simulink model "SEIRS_2_Control_Filtro"  (R2024a)
settings: Solver=VariableStepAuto  StartTime=0.0  StopTime=Dias  RelTol=1e-3
model workspace (MAT data in the model file):
  x = [0.0844291205376 0.0972801431163 0.171504041231 0.000911075297271]
undefined symbols (not defined in the file): I0, K_control, pert, R0, S0, Ts, TS, u_0, x0
libraries: simulink x1
settings Model: Creator=carlo  LastModifiedBy=luism
settings DataIOCC: SaveOutput=off
settings RTWCC: GPUComputeCapability=3.5

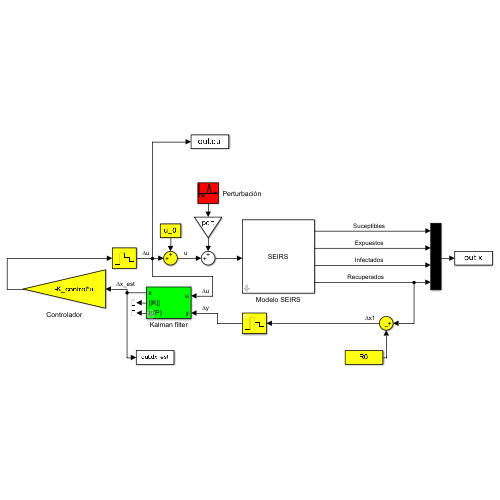
[thumbnail: Simulink's stored preview of the top-level diagram]
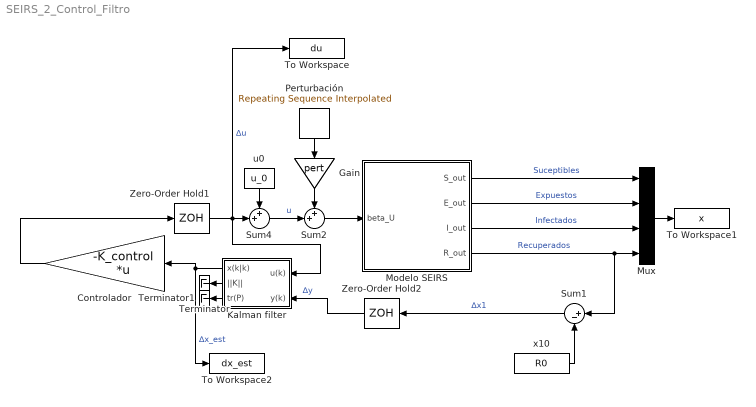
== system SEIRS_2_Control_Filtro ==
  Controlador : Gain  Gain=-K_control  Multiplication=Matrix(K*u)
  Gain : Gain  Gain=pert
  Kalman filter : Subsystem  mask(Filtro de Kalman lineal){Sd={Phi_control, Gamma_control, C_Control}, xu0=x0, P0QR={P0  Q R_k}, Ts=Ts}
      mask prompts: Sd "{A,B,C} - Discrete-time system model"; xu0 "x0 - Initial conditions"; P0QR "{P0,Q,R}"; Ts "Ts - Sample time"
      mask init:
      | A = Sd{1}; B = Sd{2}; C = Sd{3};
      | P0 = P0QR{1}; Q = P0QR{2}; R = P0QR{3};
      mask Display:
      | port_label('input', 1, 'u')
      | port_label('input', 2, 'y')
      | port_label('output', 1, 'x')
      | port_label('output', 2, '||K||')
      | port_label('output', 3, 'tr(P)')
  Modelo SEIRS : Subsystem  mask{B=0.0001, d=0.0001, alpha=0.1, gamma=0.1, beta=0.2, nu=0.001, ci=[S0 E0 I0 R0], Ruido=off, Var_ruido=1e-08}
      mask prompts: ci "[S0 E0 I0 R0]"; Ruido "Incluir ruido al sistema"; Var_ruido "Varianza del ruido"
      mask Display: disp('SEIRS');
  Mux : Mux
  Perturbación : simulink/Sources/Repeating Sequence Interpolated  OutValues=[0 0 -0.1 0 0 0.3 0 0 0.05 0]  TimeValues=[ 0 10 20 30 40 50 60 70 80 90]  LookUpMeth=Interpolation-Use End Values  tsamp=-1  OutMin=[]  OutMax=[]  OutDataTypeStr=double  OutputDataTypeScalingMode=double  OutDataType=fixdt(0,8)  OutScaling=2^-10
  Sum1 : Sum  Inputs=|+-
  Sum2 : Sum  Inputs=++|
  Sum4 : Sum  Inputs=++|
  Terminator : Terminator
  Terminator1 : Terminator
  To Workspace : ToWorkspace  VariableName=du  SaveFormat=Structure With Time  SampleTime=Ts
  To Workspace1 : ToWorkspace  VariableName=x  SaveFormat=Structure With Time  SampleTime=Ts
  To Workspace2 : ToWorkspace  VariableName=dx_est  SaveFormat=Structure With Time  SampleTime=Ts
  Zero-Order Hold1 : ZeroOrderHold  SampleTime=Ts
  Zero-Order Hold2 : ZeroOrderHold  SampleTime=Ts
  u0 : Constant  Value=u_0
  x10 : Constant  Value=R0
  wires:
  Modelo SEIRS/2(E_out) -> Mux/2  "Expuestos"
  Modelo SEIRS/3("I_out ") -> Mux/3  "Infectados"
  Modelo SEIRS/1(S_out) -> Mux/1  "Suceptibles"
  Modelo SEIRS/4(R_out) -> Sum1/1, Mux/4  "Recuperados"
  Kalman filter/1(x(k|k)) -> Controlador/1, To Workspace2/1  "∆x_est"
  Kalman filter/2(||K||) -> Terminator/1
  Gain/1 -> Sum2/1
  Kalman filter/3(tr(P)) -> Terminator1/1
  u0/1 -> Sum4/1
  Mux/1 -> To Workspace1/1
  Zero-Order Hold1/1 -> Kalman filter/1(u(k)), To Workspace/1, Sum4/2  "∆u"
  Zero-Order Hold2/1 -> Kalman filter/2(y(k))  "∆y"
  x10/1 -> Sum1/2
  Perturbación/1 -> Gain/1
  Sum1/1 -> Zero-Order Hold2/1  "∆x1"
  Controlador/1 -> Zero-Order Hold1/1
  Sum2/1 -> Modelo SEIRS/1(beta_U)
  Sum4/1 -> Sum2/2  "u"

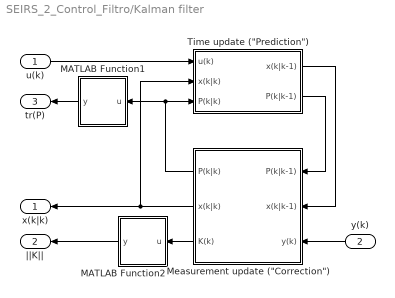
== system SEIRS_2_Control_Filtro/Kalman filter ==
  u(k) : Inport
  y(k) : Inport  Port=2
  MATLAB Function1 : MATLAB Function  TreatAsAtomicUnit=on
  MATLAB Function2 : MATLAB Function  TreatAsAtomicUnit=on
  "Measurement update (\"Correction\")" : Subsystem
  "Time update (\"Prediction\")" : Subsystem
  x(k|k) : Outport
  ||K|| : Outport  Port=2
  tr(P) : Outport  Port=3
  wires:
  MATLAB Function1/1(y) -> tr(P)/1
  MATLAB Function2/1(y) -> ||K||/1
  "Measurement update (\"Correction\")"/3(K(k)) -> MATLAB Function2/1(u)
  u(k)/1 -> "Time update (\"Prediction\")"/1(u(k))
  y(k)/1 -> "Measurement update (\"Correction\")"/3(y(k))
  "Time update (\"Prediction\")"/2(P(k|k-1)) -> "Measurement update (\"Correction\")"/1(P(k|k-1))
  "Time update (\"Prediction\")"/1(x(k|k-1)) -> "Measurement update (\"Correction\")"/2(x(k|k-1))
  "Measurement update (\"Correction\")"/2(x(k|k)) -> "Time update (\"Prediction\")"/2(x(k|k)), x(k|k)/1
  "Measurement update (\"Correction\")"/1(P(k|k)) -> "Time update (\"Prediction\")"/3(P(k|k)), MATLAB Function1/1(u)

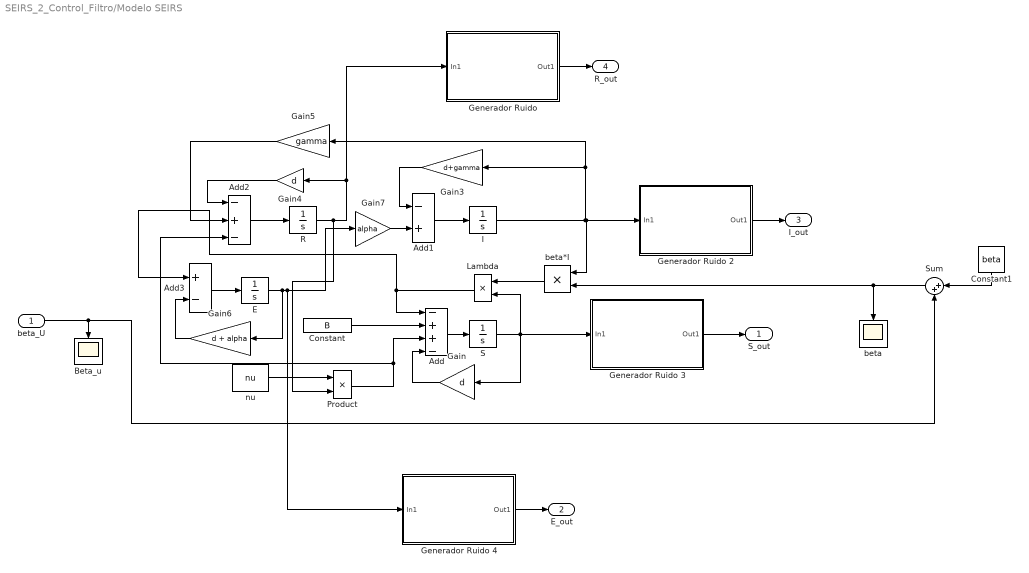
== system SEIRS_2_Control_Filtro/Modelo SEIRS ==
  beta_U : Inport
  Add : Sum  Inputs=-++-
  Add1 : Sum  Inputs=-+
  Add2 : Sum  Inputs=-+-
  Add3 : Sum  Inputs=+-
  Beta_u : Scope
  Constant : Constant  Value=B
  Constant1 : Constant  Value=beta
  E : Integrator  InitialCondition=ci(2)  LimitOutput=on  LowerSaturationLimit=0
  Gain : Gain  Gain=d
  Gain3 : Gain  Gain=d+gamma
  Gain4 : Gain  Gain=d
  Gain5 : Gain  Gain=gamma
  Gain6 : Gain  Gain=d + alpha
  Gain7 : Gain  Gain=alpha
  "Generador Ruido " : Subsystem
      mask Display: disp('Generador Ruido');
  Generador Ruido 2 : Subsystem
      mask Display: disp('Generador Ruido');
  Generador Ruido 3 : Subsystem
      mask Display: disp('Generador Ruido');
  Generador Ruido 4 : Subsystem
      mask Display: disp('Generador Ruido');
  I : Integrator  InitialCondition=ci(3)  LimitOutput=on  LowerSaturationLimit=0
  Lambda : Product
  Product : Product
  R : Integrator  InitialCondition=ci(4)  LimitOutput=on  LowerSaturationLimit=0
  S : Integrator  InitialCondition=ci(1)  LimitOutput=on  LowerSaturationLimit=0
  Sum : Sum  Inputs=|++
  beta : Scope
  beta*I : Product
  nu : Constant  Value=nu
  S_out : Outport
  E_out : Outport  Port=2
  "I_out " : Outport  Port=3
  R_out : Outport  Port=4
  wires:
  Gain/1 -> Add/4
  Gain4/1 -> Add2/1
  Constant/1 -> Add/2
  I/1 -> Generador Ruido 2/1(In1), beta*I/1, Gain5/1, Gain3/1
  Lambda/1 -> Add3/1, Add/1
  Add/1 -> S/1
  E/1 -> Gain7/1, Generador Ruido 4/1(In1), Gain6/1
  S/1 -> Generador Ruido 3/1(In1), Lambda/2, Gain/1
  Add3/1 -> E/1
  Gain3/1 -> Add1/1
  Gain5/1 -> Add2/2
  Gain6/1 -> Add3/2
  Add1/1 -> I/1
  R/1 -> "Generador Ruido "/1(In1), Gain4/1, Product/2
  Add2/1 -> R/1
  Product/1 -> Add2/3, Add/3
  Gain7/1 -> Add1/2
  nu/1 -> Product/1
  beta*I/1 -> Lambda/1
  Sum/1 -> beta*I/2, beta/1
  Constant1/1 -> Sum/1
  beta_U/1 -> Sum/2, Beta_u/1
  Generador Ruido 2/1(Out1) -> "I_out "/1
  "Generador Ruido "/1(Out1) -> R_out/1
  Generador Ruido 3/1(Out1) -> S_out/1
  Generador Ruido 4/1(Out1) -> E_out/1

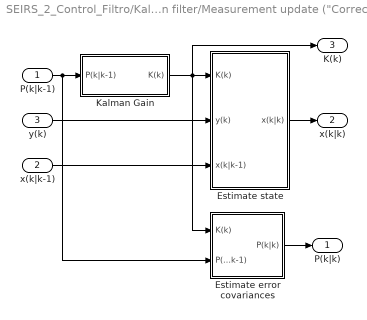
== system SEIRS_2_Control_Filtro/Kalman filter/Measurement update ("Correction") ==
  P(k|k-1) : Inport
  x(k|k-1) : Inport  Port=2
  y(k) : Inport  Port=3
  Estimate error covariances : Subsystem
  Estimate state : Subsystem
  Kalman Gain : Subsystem
  P(k|k) : Outport
  x(k|k) : Outport  Port=2
  K(k) : Outport  Port=3
  wires:
  P(k|k-1)/1 -> Kalman Gain/1(P(k|k-1)), Estimate error covariances/2(P(k|k-1))
  Kalman Gain/1(K(k)) -> Estimate state/1(K(k)), Estimate error covariances/1(K(k)), K(k)/1
  y(k)/1 -> Estimate state/2(y(k))
  Estimate state/1(x(k|k)) -> x(k|k)/1
  Estimate error covariances/1(P(k|k)) -> P(k|k)/1
  x(k|k-1)/1 -> Estimate state/3(x(k|k-1))

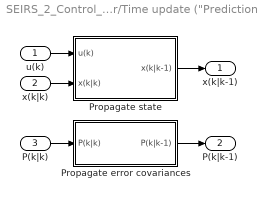
== system SEIRS_2_Control_Filtro/Kalman filter/Time update ("Prediction") ==
  u(k) : Inport
  x(k|k) : Inport  Port=2
  P(k|k) : Inport  Port=3
  Propagate error covariances : Subsystem
  Propagate state : Subsystem
  x(k|k-1) : Outport
  P(k|k-1) : Outport  Port=2
  wires:
  u(k)/1 -> Propagate state/1(u(k))
  Propagate state/1(x(k|k-1)) -> x(k|k-1)/1
  x(k|k)/1 -> Propagate state/2(x(k|k))
  P(k|k)/1 -> Propagate error covariances/1(P(k|k))
  Propagate error covariances/1(P(k|k-1)) -> P(k|k-1)/1

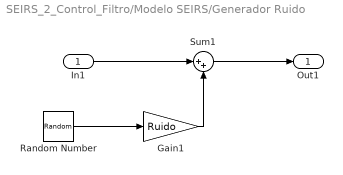
== system SEIRS_2_Control_Filtro/Modelo SEIRS/Generador Ruido  ==
  In1 : Inport
  Gain1 : Gain  Gain=Ruido
  Random Number : RandomNumber  Variance=Var_ruido  Seed=117  SampleTime=TS
  Sum1 : Sum  Inputs=|++
  Out1 : Outport
  wires:
  Random Number/1 -> Gain1/1
  Gain1/1 -> Sum1/2
  In1/1 -> Sum1/1
  Sum1/1 -> Out1/1

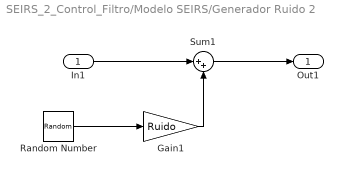
== system SEIRS_2_Control_Filtro/Modelo SEIRS/Generador Ruido 2 ==
  In1 : Inport
  Gain1 : Gain  Gain=Ruido
  Random Number : RandomNumber  Variance=Var_ruido  Seed=117  SampleTime=TS
  Sum1 : Sum  Inputs=|++
  Out1 : Outport
  wires:
  Random Number/1 -> Gain1/1
  Gain1/1 -> Sum1/2
  In1/1 -> Sum1/1
  Sum1/1 -> Out1/1

== system SEIRS_2_Control_Filtro/Modelo SEIRS/Generador Ruido 3 ==
  In1 : Inport
  Gain1 : Gain  Gain=Ruido
  Random Number : RandomNumber  Variance=Var_ruido  Seed=117  SampleTime=TS
  Sum1 : Sum  Inputs=|++
  Out1 : Outport
  wires:
  Random Number/1 -> Gain1/1
  Gain1/1 -> Sum1/2
  In1/1 -> Sum1/1
  Sum1/1 -> Out1/1

== system SEIRS_2_Control_Filtro/Modelo SEIRS/Generador Ruido 4 ==
  In1 : Inport
  Gain1 : Gain  Gain=Ruido
  Random Number : RandomNumber  Variance=Var_ruido  Seed=117  SampleTime=TS
  Sum1 : Sum  Inputs=|++
  Out1 : Outport
  wires:
  Random Number/1 -> Gain1/1
  Gain1/1 -> Sum1/2
  In1/1 -> Sum1/1
  Sum1/1 -> Out1/1

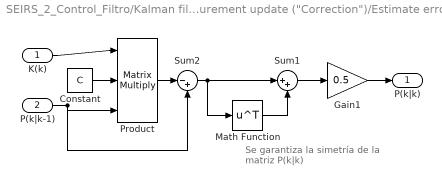
== system SEIRS_2_Control_Filtro/Kalman filter/Measurement update ("Correction")/Estimate error covariances ==
  note: Se garantiza la simetría
      | de la matriz P(k|k)
  K(k) : Inport
  P(k|k-1) : Inport  Port=2
  Constant : Constant  Value=C  VectorParams1D=off  SampleTime=Ts
  Gain1 : Gain  Gain=0.5
  Math Function : Math  Operator=transpose  SignedPower=on
  Product : Product  Inputs=3  Multiplication=Matrix(*)
  Sum1 : Sum  Inputs=|++
  Sum2 : Sum  Inputs=|-+
  P(k|k) : Outport
  wires:
  Constant/1 -> Product/2
  Product/1 -> Sum2/1
  K(k)/1 -> Product/1
  P(k|k-1)/1 -> Sum2/2, Product/3
  Gain1/1 -> P(k|k)/1
  Sum2/1 -> Math Function/1, Sum1/1
  Math Function/1 -> Sum1/2
  Sum1/1 -> Gain1/1

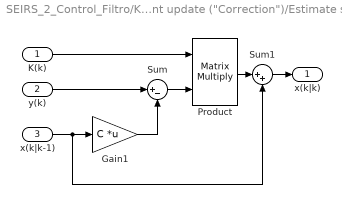
== system SEIRS_2_Control_Filtro/Kalman filter/Measurement update ("Correction")/Estimate state ==
  K(k) : Inport
  y(k) : Inport  Port=2
  x(k|k-1) : Inport  Port=3
  Gain1 : Gain  Gain=C  Multiplication=Matrix(K*u)
  Product : Product  Multiplication=Matrix(*)
  Sum : Sum  Inputs=|+-
  Sum1 : Sum  Inputs=|++
  x(k|k) : Outport
  wires:
  x(k|k-1)/1 -> Sum1/2, Gain1/1
  Gain1/1 -> Sum/2
  Sum/1 -> Product/2
  Product/1 -> Sum1/1
  K(k)/1 -> Product/1
  Sum1/1 -> x(k|k)/1
  y(k)/1 -> Sum/1

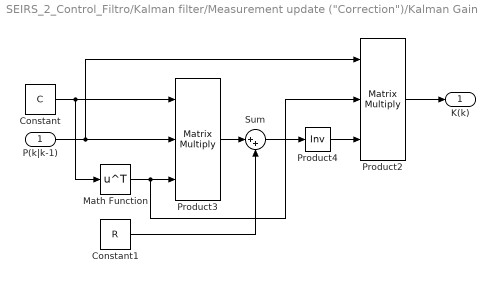
== system SEIRS_2_Control_Filtro/Kalman filter/Measurement update ("Correction")/Kalman Gain ==
  P(k|k-1) : Inport
  Constant : Constant  Value=C  VectorParams1D=off  SampleTime=Ts
  Constant1 : Constant  Value=R  SampleTime=Ts
  Math Function : Math  Operator=transpose  SignedPower=on
  Product2 : Product  Inputs=3  Multiplication=Matrix(*)
  Product3 : Product  Inputs=3  Multiplication=Matrix(*)
  Product4 : Product  Inputs=/  Multiplication=Matrix(*)
  Sum : Sum  Inputs=|++
  K(k) : Outport
  wires:
  Constant/1 -> Math Function/1, Product3/1
  P(k|k-1)/1 -> Product3/2, Product2/1
  Math Function/1 -> Product3/3, Product2/2
  Product3/1 -> Sum/1
  Constant1/1 -> Sum/2
  Sum/1 -> Product4/1
  Product4/1 -> Product2/3
  Product2/1 -> K(k)/1

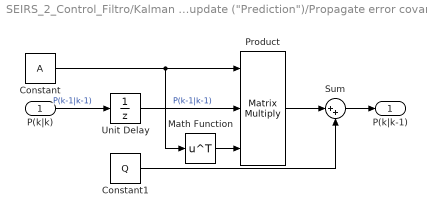
== system SEIRS_2_Control_Filtro/Kalman filter/Time update ("Prediction")/Propagate error covariances ==
  P(k|k) : Inport
  Constant : Constant  Value=A  SampleTime=Ts
  Constant1 : Constant  Value=Q  SampleTime=Ts
  Math Function : Math  Operator=transpose  SignedPower=on
  Product : Product  Inputs=3  Multiplication=Matrix(*)  RndMeth=Zero  SampleTime=Ts
  Sum : Sum  Inputs=|++
  Unit Delay : UnitDelay  InitialCondition=P0  SampleTime=Ts  HasFrameUpgradeWarning=on
  P(k|k-1) : Outport
  wires:
  P(k|k)/1 -> Unit Delay/1  "P(k-1|k-1)"
  Constant/1 -> Math Function/1, Product/1
  Math Function/1 -> Product/3
  Product/1 -> Sum/1
  Constant1/1 -> Sum/2
  Sum/1 -> P(k|k-1)/1
  Unit Delay/1 -> Product/2  "P(k-1|k-1)"

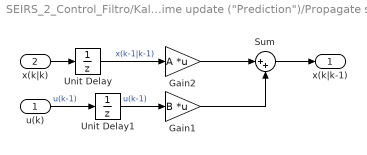
== system SEIRS_2_Control_Filtro/Kalman filter/Time update ("Prediction")/Propagate state ==
  u(k) : Inport
  x(k|k) : Inport  Port=2
  Gain1 : Gain  Gain=B  Multiplication=Matrix(K*u)
  Gain2 : Gain  Gain=A  Multiplication=Matrix(K*u)
  Sum : Sum  Inputs=|++
  Unit Delay : UnitDelay  InitialCondition=x0  SampleTime=Ts  HasFrameUpgradeWarning=on
  Unit Delay1 : UnitDelay  SampleTime=Ts  HasFrameUpgradeWarning=on
  x(k|k-1) : Outport
  wires:
  Unit Delay/1 -> Gain2/1  "x(k-1|k-1)"
  x(k|k)/1 -> Unit Delay/1
  u(k)/1 -> Unit Delay1/1  "u(k-1)"
  Gain2/1 -> Sum/1
  Gain1/1 -> Sum/2
  Sum/1 -> x(k|k-1)/1
  Unit Delay1/1 -> Gain1/1  "u(k-1)"

== matlab function SEIRS_2_Control_Filtro/Kalman filter/MATLAB Function1 ==
  data: u input; y output
function y = fcn(u)
y = trace(u);

== matlab function SEIRS_2_Control_Filtro/Kalman filter/MATLAB Function2 ==
  data: u input; y output
function y = fcn(u)
y = norm(u);
